simulink model "NewTRy"  (R2019b)
settings: Solver=VariableStepAuto  StartTime=0.0  StopTime=10.0  RelTol=1e-3
values from neighbouring files (symbols this model uses):
  alpha = J + (M + (1/3)*ma + mp)*la^2    (= 0.000202475)    [InitEqVerify.m]    (also in NewTryInit.m)
  beta = (M + (1/3)*mp)*lp^2    (= 7.05159e-06)    [InitEqVerify.m]    (also in NewTryInit.m)
  delta = (M + (1/2)*mp)*g*lp    (= 0.002451078)    [InitEqVerify.m]    (also in NewTryInit.m)
  gamma = (M + (1/2)*mp)*la*lp    (= 1.875825e-05)    [InitEqVerify.m]    (also in NewTryInit.m)
settings Model: Creator=trulsmartinsson  LastModifiedBy=trulsmartinsson

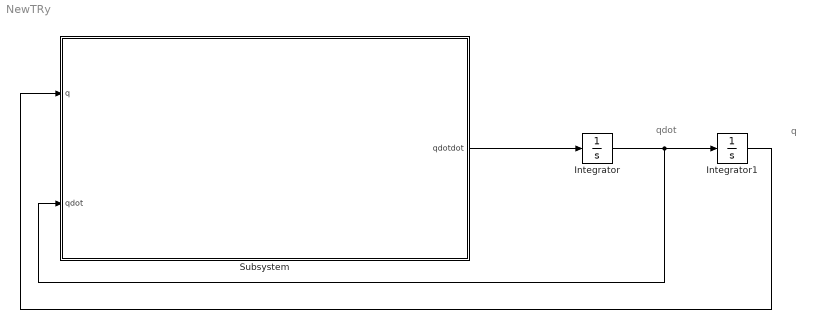
== system NewTRy ==
  note: q
  note: qdot
  Integrator : Integrator
  Integrator1 : Integrator
  Subsystem : Subsystem
  wires:
  Subsystem/1("qdotdot ") -> Integrator/1
  Integrator/1 -> Subsystem/2("qdot "), Integrator1/1
  Integrator1/1 -> Subsystem/1("q ")

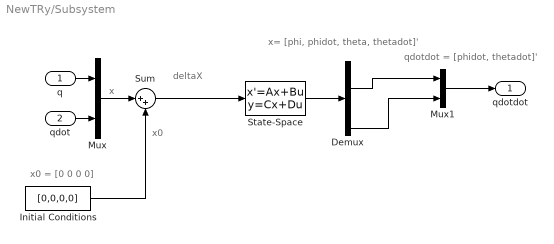
== system NewTRy/Subsystem ==
  note: x= [phi, phidot, theta, thetadot]'
  note: qdotdot = [phidot, thetadot]'
  note: x0 = [0 0 0 0]
  note: x0
  note: x
  note: deltaX
  "q " : Inport
  "qdot " : Inport  Port=2
  Demux : Demux
  "Initial Conditions " : FromWorkspace  VariableName=[0,0,0,0]  SampleTime=0
  Mux : Mux  Inputs=2
  Mux1 : Mux  Inputs=2
  State-Space : StateSpace  A=[0,1,0,0; 0,0, -((delta*gamma)/((alpha*beta - gamma^2))), 0; 0,0,0,1; 0,0, ((alpha*delta)/((alpha*beta) - gamma^2)),0]  B=[0,0; ((beta)/((alpha*beta) - gamma^2)), -((gamma)/((alpha*beta) - gamma^2)) ;0,0; -(gamma/((alpha*beta)- gamma^2)), (alpha/((alpha*beta)-gamma^2)) ]  C=[0,0,0,0]  D=[0,0]  InitialCondition=0
  Sum : Sum  Inputs=|++
  "qdotdot " : Outport
  wires:
  "q "/1 -> Mux/1
  "qdot "/1 -> Mux/2
  Mux/1 -> Sum/1
  "Initial Conditions "/1 -> Sum/2
  State-Space/1 -> Demux/1
  Demux/2 -> Mux1/1
  Demux/4 -> Mux1/2
  Mux1/1 -> "qdotdot "/1
  Sum/1 -> State-Space/1
